simulink model "chassis"  (R2021b)
settings: Solver=VariableStepAuto  StartTime=0.0  StopTime=10.0  RelTol=1e-3
settings Model: Creator=Geton  LastModifiedBy=Geton

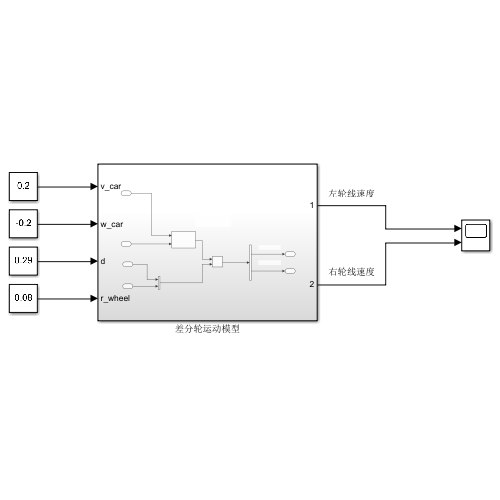
[thumbnail: Simulink's stored preview of the top-level diagram]
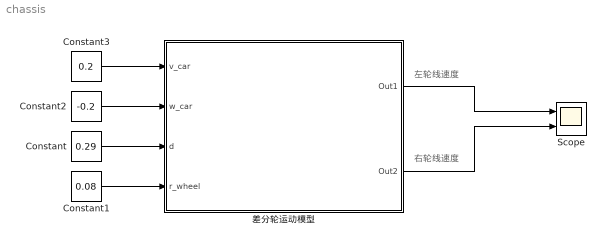
== system chassis ==
  note: 右轮线速度
  note: 左轮线速度
  Constant : Constant  Value=0.29
  Constant1 : Constant  Value=0.08
  Constant2 : Constant  Value=-0.2
  Constant3 : Constant  Value=0.2
  Scope : Scope  NumInputPorts=2
  差分轮运动模型 : Subsystem
  wires:
  Constant/1 -> 差分轮运动模型/3(d)
  Constant1/1 -> 差分轮运动模型/4(r_wheel)
  Constant2/1 -> 差分轮运动模型/2(w_car)
  Constant3/1 -> 差分轮运动模型/1(v_car)
  差分轮运动模型/1(Out1) -> Scope/1
  差分轮运动模型/2(Out2) -> Scope/2

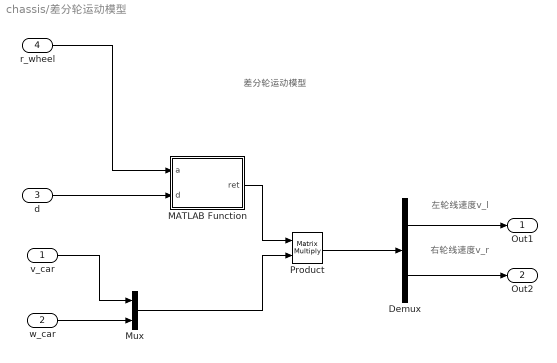
== system chassis/差分轮运动模型 ==
  note: 左轮线速度v_l
  note: 差分轮运动模型
  note: 右轮线速度v_r
  v_car : Inport
  w_car : Inport  Port=2
  d : Inport  Port=3
  r_wheel : Inport  Port=4
  Demux : Demux  Outputs=2
  MATLAB Function : MATLAB Function  TreatAsAtomicUnit=on
  Mux : Mux  Inputs=2
  Product : Product  Multiplication=Matrix(*)
  Out1 : Outport
  Out2 : Outport  Port=2
  wires:
  v_car/1 -> Mux/1
  w_car/1 -> Mux/2
  Mux/1 -> Product/2
  r_wheel/1 -> MATLAB Function/1(a)
  d/1 -> MATLAB Function/2(d)
  MATLAB Function/1(ret) -> Product/1
  Product/1 -> Demux/1
  Demux/1 -> Out1/1
  Demux/2 -> Out2/1

== matlab function chassis/差分轮运动模型/MATLAB Function ==
  data: a input; ret output; d input
function ret = fcn(a,d)
   ret=[1/a -d/a;
       1/a  d/a];
